simulink model "adaptive_sliding_mode_control"  (R2019b)
settings: Solver=VariableStepAuto  StartTime=0  StopTime=5  RelTol=1e-3
settings Model: Creator=Alien  LastModifiedBy=Alien

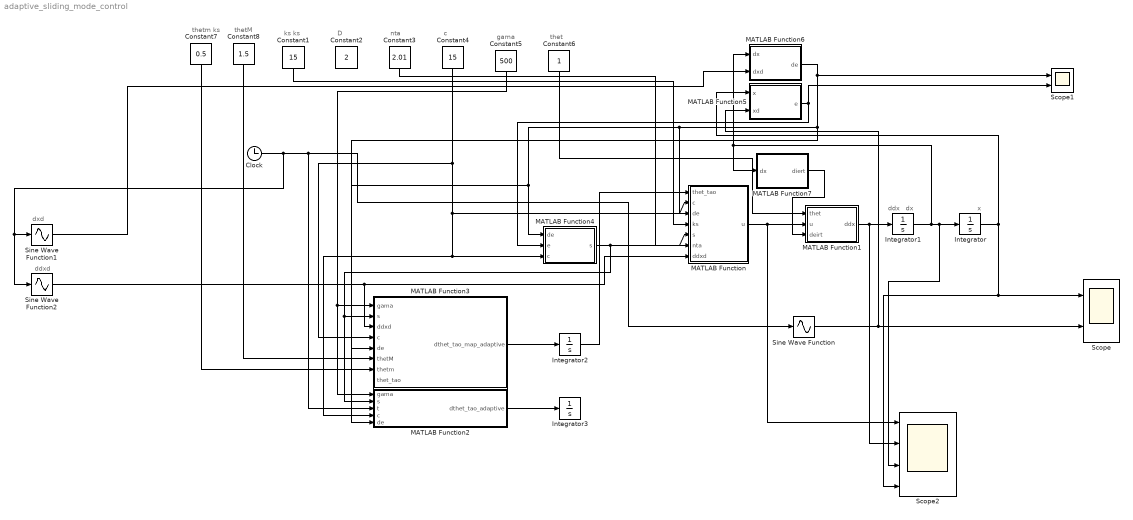
== system adaptive_sliding_mode_control ==
  note: ddxd
  note: dxd
  note: ddx
  note: dx
  note: x
  note: nta
  note: c
  note: D
  note: ks
      | ks
  note: thet
  note: gama
  note: thetm
      | ks
  note: thetM
  Clock : Clock
  Constant1 : Constant  Value=15
  Constant2 : Constant  Value=2
  Constant3 : Constant  Value=2.01
  Constant4 : Constant  Value=15
  Constant5 : Constant  Value=500
  Constant6 : Constant
  Constant7 : Constant  Value=0.5
  Constant8 : Constant  Value=1.5
  Integrator : Integrator  InitialCondition=6
  Integrator1 : Integrator  InitialCondition=2
  Integrator2 : Integrator  InitialCondition=1
  Integrator3 : Integrator
  MATLAB Function : MATLAB Function  TreatAsAtomicUnit=on
  MATLAB Function1 : MATLAB Function  TreatAsAtomicUnit=on
  MATLAB Function2 : MATLAB Function  TreatAsAtomicUnit=on
  MATLAB Function3 : MATLAB Function  TreatAsAtomicUnit=on
  MATLAB Function4 : MATLAB Function  TreatAsAtomicUnit=on
  MATLAB Function5 : MATLAB Function  TreatAsAtomicUnit=on
  MATLAB Function6 : MATLAB Function  TreatAsAtomicUnit=on
  MATLAB Function7 : MATLAB Function  TreatAsAtomicUnit=on
  Scope : Scope  NumInputPorts=2
  Scope1 : Scope  NumInputPorts=2
  Scope2 : Scope  NumInputPorts=4
  Sine Wave Function : Sin  TimeSource=Use external signal  SampleTime=0
  Sine Wave Function1 : Sin  TimeSource=Use external signal  Phase=pi/2  SampleTime=0
  Sine Wave Function2 : Sin  TimeSource=Use external signal  Amplitude=-1  SampleTime=0
  wires:
  Integrator1/1 -> MATLAB Function6/1(dx), MATLAB Function7/1(dx), Scope2/3, Integrator/1
  MATLAB Function1/1(ddx) -> Scope2/2, Integrator1/1
  MATLAB Function3/1(dthet_tao_map_adaptive) -> Integrator2/1
  Integrator/1 -> Scope2/4, Scope/1, MATLAB Function5/1(x)
  MATLAB Function2/1(dthet_tao_adaptive) -> Integrator3/1
  MATLAB Function/1(u) -> Scope2/1, MATLAB Function1/2(u)
  MATLAB Function7/1(diert) -> MATLAB Function1/3(deirt)
  MATLAB Function4/1(s) -> MATLAB Function3/2(s), MATLAB Function2/2(s), MATLAB Function/5(s)
  MATLAB Function6/1(de) -> MATLAB Function3/5(de), MATLAB Function/3(de), MATLAB Function2/5(de), MATLAB Function4/1(de), Scope1/1
  MATLAB Function5/1(e) -> MATLAB Function4/2(e), Scope1/2
  Constant4/1 -> MATLAB Function3/4(c), MATLAB Function/2(c), MATLAB Function2/4(c), MATLAB Function4/3(c)
  Clock/1 -> Sine Wave Function2/1, Sine Wave Function1/1, MATLAB Function2/3(t), Sine Wave Function/1
  Constant6/1 -> MATLAB Function1/1(thet)
  Constant5/1 -> MATLAB Function3/1(gama), MATLAB Function2/1(gama)
  Constant1/1 -> MATLAB Function/4(ks)
  Constant3/1 -> MATLAB Function/6(nta)
  Sine Wave Function/1 -> MATLAB Function5/2(xd), Scope/2
  Constant8/1 -> MATLAB Function3/6(thetM)
  Constant7/1 -> MATLAB Function3/7(thetm)
  Sine Wave Function2/1 -> MATLAB Function3/3(ddxd), MATLAB Function/7(ddxd)
  Sine Wave Function1/1 -> MATLAB Function6/2(dxd)
  Integrator2/1 -> MATLAB Function/1(thet_tao)

== matlab function adaptive_sliding_mode_control/MATLAB Function1 ==
  data: thet input; u input; ddx output; deirt input
function ddx = fcn(thet,u, deirt)
ddx = 1/thet*(u - deirt);

== matlab function adaptive_sliding_mode_control/MATLAB Function ==
  data: thet_tao input; c input; de input; ks input; s input; nta input; u output; ddxd input
function u = fcn(thet_tao, c, de, ks, s, nta, ddxd)
u = thet_tao*(ddxd - c*de) - ks*s - nta*sign(s);

== matlab function adaptive_sliding_mode_control/MATLAB Function2 ==
  data: gama input; dthet_tao_adaptive output; s input; t input; c input; de input
function dthet_tao_adaptive = fcn(gama, s, t, c, de)
ddxd = -sin(t);
dthet_tao_adaptive = -gama*s*(ddxd - c*de);

== matlab function adaptive_sliding_mode_control/MATLAB Function3 ==
  data: gama input; dthet_tao_map_adaptive output; s input; ddxd input; c input; de input; thetM input; thetm input; thet_tao input
function dthet_tao_map_adaptive = fcn(gama, s, ddxd, c, de, thetM, thetm, thet_tao)
dthet_tao_map_adaptive = -gama*s*(ddxd - c*de);
if(thet_tao >= thetM && dthet_tao_map_adaptive > 0)
    dthet_tao_map_adaptive = 0;
elseif(thet_tao <= thetm && dthet_tao_map_adaptive < 0)
    dthet_tao_map_adaptive = 0;
end

== matlab function adaptive_sliding_mode_control/MATLAB Function4 ==
  data: de input; s output; e input; c input
function s = fcn(de, e, c)
s = de + c*e;

== matlab function adaptive_sliding_mode_control/MATLAB Function5 ==
  data: x input; e output; xd input
function e = fcn(x, xd)
e = x - xd;

== matlab function adaptive_sliding_mode_control/MATLAB Function6 ==
  data: dx input; de output; dxd input
function de = fcn(dx, dxd)
de = dx - dxd;

== matlab function adaptive_sliding_mode_control/MATLAB Function7 ==
  data: dx input; diert output
function diert = fcn(dx)
diert = dx/2 + 1.5*sign(dx);
